simulink model "adaptive_motor_sim"  (R2025b)
settings: Solver=FixedStepDiscrete  StartTime=0.0  StopTime=simTime  FixedStep=T  RelTol=1e-3
InitFcn:
  | run(fullfile(fileparts(get_param(bdroot,'FileName')), 'adaptive_motor_params.m'));
values from neighbouring files (symbols this model uses):
  alpha = 0.98    [adaptive_motor_params.m]    (also in identifiability_study.m = 1)
  b = 1    [adaptive_motor_params.m]    (also in export_sim_plots.m = 0.0005; validate_stage_models.m)
  b0Min = 1e-3    (= 0.001)    [adaptive_motor_params.m]
  J_large = 24    [adaptive_motor_params.m]    (also in validate_stage_models.m)
  J_small = 1    [adaptive_motor_params.m]    (also in validate_stage_models.m)
  Km = 1    [adaptive_motor_params.m]    (also in export_sim_plots.m = 0.05; validate_stage_models.m)
  noiseSeed = 23341    [adaptive_motor_params.m]
  noiseVariance = 1e-3 / T    (= 0.0125)    [adaptive_motor_params.m]
  q0 = 0.06    [adaptive_motor_params.m]    (also in export_sim_plots.m)
  q1 = -0.5    [adaptive_motor_params.m]    (also in export_sim_plots.m)
  refAmplitude = 50    [adaptive_motor_params.m]
  refPeriod = 16    [adaptive_motor_params.m]
  swapTime = 32    [adaptive_motor_params.m]
  T = 0.08    [adaptive_motor_params.m]    (also in build_second_order_model.m = num(p.T); build_stage_models.m = num(p.T); export_sim_plots.m; validate_stage_models.m)
  uMax = 255    [adaptive_motor_params.m]    (also in validate_stage_models.m)
  uMin = -255    [adaptive_motor_params.m]
settings Model: Creator=Lenard  LastModifiedBy=Lenard

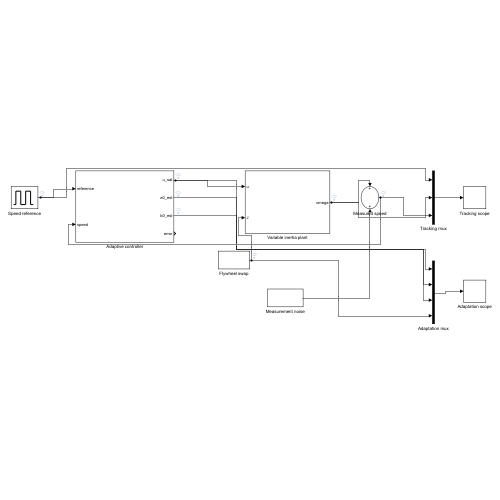
[thumbnail: Simulink's stored preview of the top-level diagram]
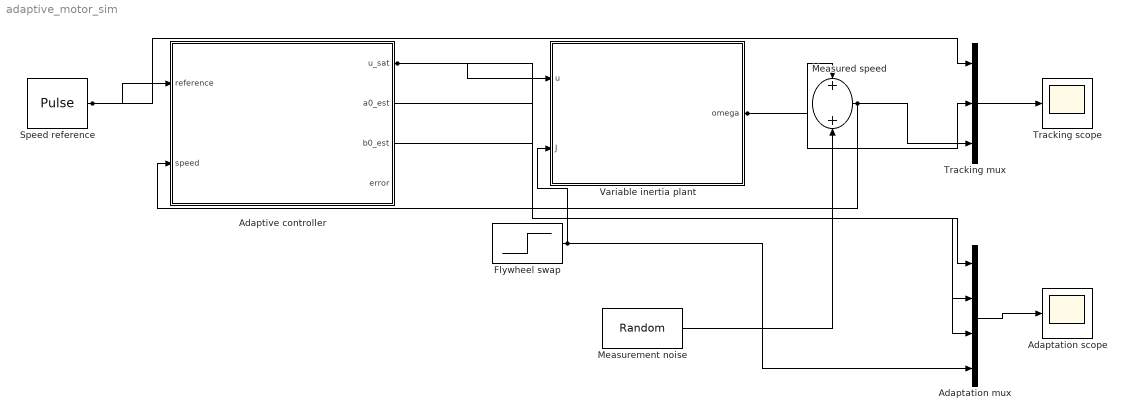
== system adaptive_motor_sim ==
  Adaptation mux : Mux
  Adaptation scope : Scope
  Adaptive controller : Subsystem
  Flywheel swap : Step  Time=swapTime  Before=J_small  After=J_large  SampleTime=T
  Measured speed : Sum
  Measurement noise : RandomNumber  Variance=noiseVariance  Seed=noiseSeed  SampleTime=T
  Speed reference : DiscretePulseGenerator  PulseType=Time based  Amplitude=refAmplitude  Period=refPeriod  PulseWidth=50  SampleTime=T
  Tracking mux : Mux  Inputs=3
  Tracking scope : Scope
  Variable inertia plant : Subsystem
  wires:
  Speed reference/1 -> Adaptive controller/1(reference), Tracking mux/1
  Adaptive controller/1(u_sat) -> Variable inertia plant/1(u), Adaptation mux/1
  Flywheel swap/1 -> Variable inertia plant/2(J), Adaptation mux/4
  Variable inertia plant/1(omega) -> Measured speed/1, Tracking mux/2
  Measurement noise/1 -> Measured speed/2
  Measured speed/1 -> Adaptive controller/2(speed), Tracking mux/3
  Tracking mux/1 -> Tracking scope/1
  Adaptive controller/2(a0_est) -> Adaptation mux/2
  Adaptive controller/3(b0_est) -> Adaptation mux/3
  Adaptation mux/1 -> Adaptation scope/1

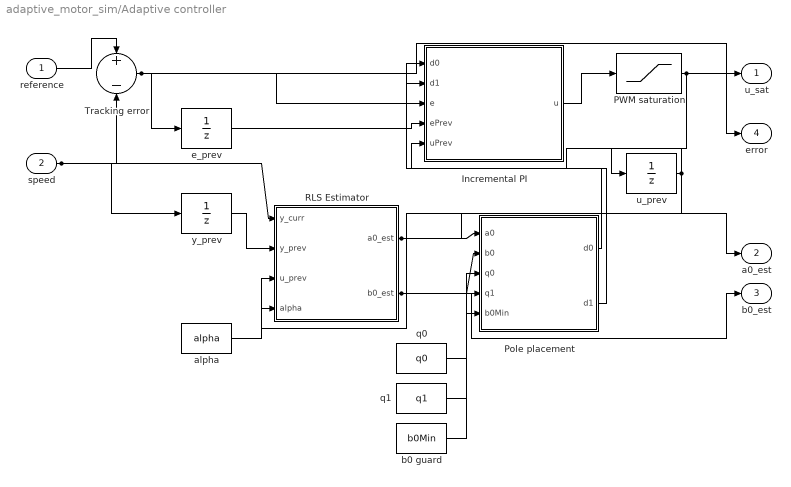
== system adaptive_motor_sim/Adaptive controller ==
  reference : Inport
  speed : Inport  Port=2
  Incremental PI : MATLAB Function  TreatAsAtomicUnit=on
  PWM saturation : Saturate  UpperLimit=uMax  LowerLimit=uMin
  Pole placement : MATLAB Function  TreatAsAtomicUnit=on
  RLS Estimator : MATLAB Function  TreatAsAtomicUnit=on
  Tracking error : Sum  Inputs=+-
  alpha : Constant  Value=alpha
  b0 guard : Constant  Value=b0Min
  e_prev : UnitDelay  SampleTime=T  HasFrameUpgradeWarning=on
  q0 : Constant  Value=q0
  q1 : Constant  Value=q1
  u_prev : UnitDelay  SampleTime=T  HasFrameUpgradeWarning=on
  y_prev : UnitDelay  SampleTime=T  HasFrameUpgradeWarning=on
  u_sat : Outport
  a0_est : Outport  Port=2
  b0_est : Outport  Port=3
  error : Outport  Port=4
  wires:
  reference/1 -> Tracking error/1
  speed/1 -> Tracking error/2, y_prev/1, RLS Estimator/1(y_curr)
  Tracking error/1 -> e_prev/1, Incremental PI/3(e), error/1
  y_prev/1 -> RLS Estimator/2(y_prev)
  u_prev/1 -> RLS Estimator/3(u_prev), Incremental PI/5(uPrev)
  alpha/1 -> RLS Estimator/4(alpha)
  RLS Estimator/1(a0_est) -> Pole placement/1(a0), a0_est/1
  RLS Estimator/2(b0_est) -> Pole placement/2(b0), b0_est/1
  q0/1 -> Pole placement/3(q0)
  q1/1 -> Pole placement/4(q1)
  b0 guard/1 -> Pole placement/5(b0Min)
  Pole placement/1(d0) -> Incremental PI/1(d0)
  Pole placement/2(d1) -> Incremental PI/2(d1)
  e_prev/1 -> Incremental PI/4(ePrev)
  Incremental PI/1(u) -> PWM saturation/1
  PWM saturation/1 -> u_prev/1, u_sat/1

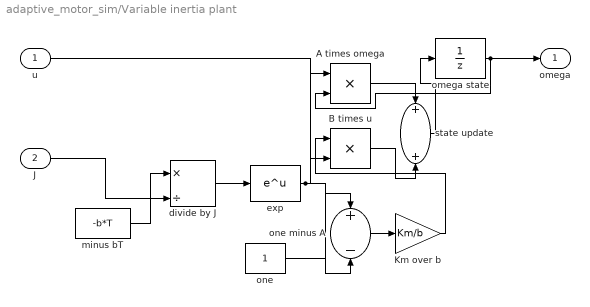
== system adaptive_motor_sim/Variable inertia plant ==
  u : Inport
  J : Inport  Port=2
  A times omega : Product
  B times u : Product
  Km over b : Gain  Gain=Km/b
  divide by J : Product  Inputs=*/
  exp : Math
  minus bT : Constant  Value=-b*T
  omega state : UnitDelay  SampleTime=T  HasFrameUpgradeWarning=on
  one : Constant
  one minus A : Sum  Inputs=+-
  state update : Sum
  omega : Outport
  wires:
  J/1 -> divide by J/2
  minus bT/1 -> divide by J/1
  divide by J/1 -> exp/1
  exp/1 -> one minus A/2, A times omega/1
  one/1 -> one minus A/1
  one minus A/1 -> Km over b/1
  omega state/1 -> A times omega/2, omega/1
  Km over b/1 -> B times u/1
  u/1 -> B times u/2
  A times omega/1 -> state update/1
  B times u/1 -> state update/2
  state update/1 -> omega state/1

== matlab function adaptive_motor_sim/Adaptive controller/Pole placement ==
  data: a0 input; d0 output; b0 input; q0 input; q1 input; b0Min input; d1 output
function [d0,d1] = pole_placement(a0,b0,q0,q1,b0Min)
                                                   %#codegen                                           
                                                   persistent d0Hold d1Hold                            
                                                   if isempty(d0Hold)                                  
                                                       d0Hold = -0.44;                                 
                                                       d1Hold = 1.0;                                   
                                                   end                                                 
                                                   if abs(b0) > b0Min                                  
                                                       d0Hold = (q0 + a0) / b0;                        
                                                       d1Hold = (q1 + 1.0 - a0) / b0;                  
                                                   end                                                 
                                                   d0 = d0Hold;                                        
                                                   d1 = d1Hold;                                        
                                                   end

== matlab function adaptive_motor_sim/Adaptive controller/RLS Estimator ==
  data: y_curr input; a0_est output; y_prev input; u_prev input; alpha input; b0_est output
function [a0_est,b0_est] = rls_estimator(y_curr,y_prev,u_prev,alpha)
                                                                   %#codegen                                                           
                                                                   persistent P xe                                                     
                                                                   if isempty(P)                                                       
                                                                       P = 100.0 * eye(2);                                             
                                                                       xe = [-0.5; 1.0];                                               
                                                                   end                                                                 
                                                                   C = [-y_prev, u_prev];                                              
                                                                   den = C * P * C' + alpha;                                           
                                                                   L = (P * C') / den;                                                 
                                                                   xe = xe + L * (y_curr - C * xe);                                    
                                                                   P = (eye(2) - L * C) * P / alpha;                                   
                                                                   P = 0.5 * (P + P');                                                 
                                                                   a0_est = xe(1);                                                     
                                                                   b0_est = xe(2);                                                     
                                                                   end

== matlab function adaptive_motor_sim/Adaptive controller/Incremental PI ==
  data: d0 input; u output; d1 input; e input; ePrev input; uPrev input
function u = incremental_pi(d0,d1,e,ePrev,uPrev)
                                               %#codegen                                       
                                               u = uPrev + d1 * e + d0 * ePrev;                
                                               end
